simulink model "FrameStructTest"  (R2022b)
settings: Solver=VariableStepAuto  StartTime=0.0  StopTime=0.01  RelTol=1e-3
model workspace (MAT data in the model file):
  f_s : Simulink.Parameter (value not decoded)
symbols that are objects in the model workspace (value not decoded): f_s
libraries: simulink x24, hdlsllib x14, dspsigops x8, commdigbbndapm x3, dsphdlfiltering2 x2, commfilt2 x2, commdigbbndpm3 x2, commrandsrc3 x1
(part 2 of 2)

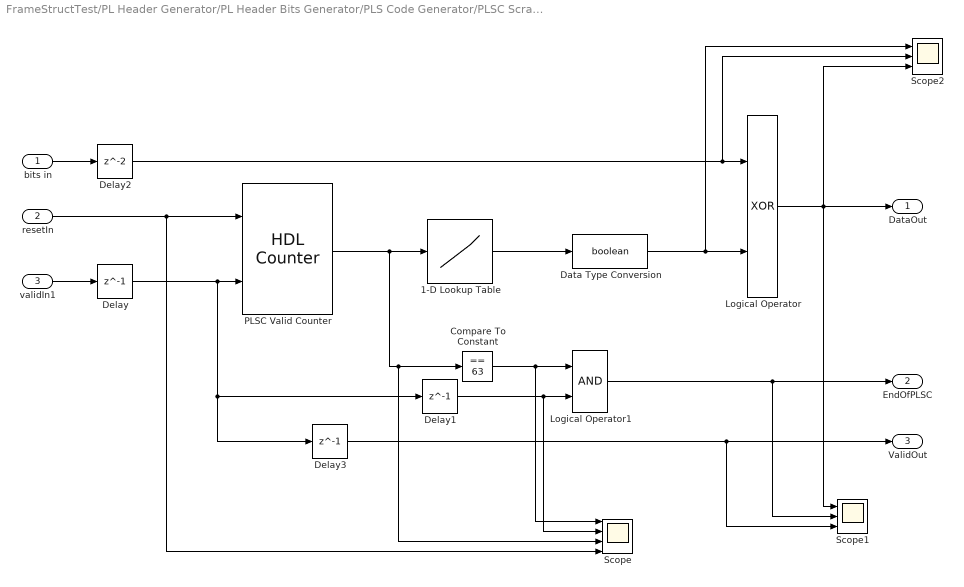
== system FrameStructTest/PL Header Generator/PL Header Bits Generator/PLS Code Generator/PLSC Scrambler ==
  bits in : Inport
  resetIn : Inport  Port=2
  validIn1 : Inport  Port=3
  1-D Lookup Table : Lookup_n-D  NumberOfTableDimensions=1  LookupTableObject=''  BreakpointsSpecification=Even spacing  BreakpointsForDimension1=[-5:5]  BreakpointsForDimension1FirstPoint=0  BreakpointsForDimension2FirstPoint=10  BreakpointsForDimension2Spacing=12  IndexSearchMethod=Evenly spaced points  Table=[1 0 1 1 1 1 0 0 0 0 0 1 0 0 0 1 1 0 0 0 0 0 0 0 1 0 1 0 0 1 0 1 0 1 0 1 0 0 0 1 0 1 1 1 0 1 1 1 0 1 0 1 1 1 0 0 1 0 0 1 1 1 0 1 1 0 0 0 0 1 0 1 1 0 0 0 1 1 1 1 1 1 0 1 1 0 1 0 1 1 0 0 1 1 0 1 1 0 1 1 1 0 0 0 0 1 1 1 0 0 0 1 1 0 1 0 1 0 0 1 1 1 1 1 0 0 0 1 0 0 0 0 1 1 0 0 1 0 1 0 0 0 0 0 0 1 1 1 1 0 1 1 1 1]  InterpMethod=Flat  DiagnosticForOutOfRangeInput=Error  InternalRulePriority=Speed  RndMeth=Simplest
  Compare To Constant : simulink/Logic and Bit Operations/Compare To Constant  relop===  const=63  OutDataTypeStr=boolean
  Data Type Conversion : DataTypeConversion  OutDataTypeStr=boolean  SaturateOnIntegerOverflow=off  RndMeth=Floor
  Delay : Delay  DelayLength=1
  Delay1 : Delay  DelayLength=1
  Delay2 : Delay
  Delay3 : Delay  DelayLength=1
  Logical Operator : Logic  Operator=XOR  AllPortsSameDT=off  OutDataTypeStr=boolean
  Logical Operator1 : Logic  AllPortsSameDT=off  OutDataTypeStr=boolean
  PLSC Valid Counter : hdlsllib/Sources/HDL Counter  CountType=Count limited  CountInit=0  CountStep=1  CountMax=154-1  CountFromType=Initial value  CountFrom=0  CountResetPort=on  CountLoadPort=off  CountEnbPort=on  CountDirPort=off  CountHitOutputPort=off  CountDataType=Unsigned  CountWordLen=8  CountFracLen=0  CountSampTime=1
  Scope : Scope  NumInputPorts=4
  Scope1 : Scope  NumInputPorts=3
  Scope2 : Scope  NumInputPorts=3
  DataOut : Outport
  EndOfPLSC : Outport  Port=2
  ValidOut : Outport  Port=3
  wires:
  PLSC Valid Counter/1 -> Scope/3, Compare To Constant/1, 1-D Lookup Table/1
  Data Type Conversion/1 -> Scope2/1, Logical Operator/2
  Logical Operator1/1 -> Scope1/2, EndOfPLSC/1
  Logical Operator/1 -> Scope2/3, Scope1/1, DataOut/1
  validIn1/1 -> Delay/1
  resetIn/1 -> Scope/4, PLSC Valid Counter/1
  Delay/1 -> Delay1/1, Delay3/1, PLSC Valid Counter/2
  Compare To Constant/1 -> Scope/1, Logical Operator1/1
  Delay1/1 -> Scope/2, Logical Operator1/2
  bits in/1 -> Delay2/1
  1-D Lookup Table/1 -> Data Type Conversion/1
  Delay2/1 -> Scope2/2, Logical Operator/1
  Delay3/1 -> Scope1/3, ValidOut/1

== system FrameStructTest/PL Header Generator/PL Header Bits Generator/PLS Code Generator/Serializer ==
  trigger : Inport
  coded bits : Inport  Port=2
  Compare To Constant : simulink/Logic and Bit Operations/Compare To Constant  relop===  const=1  OutDataTypeStr=boolean
  Compare To Constant1 : simulink/Logic and Bit Operations/Compare To Constant  relop=~=  const=1  OutDataTypeStr=boolean
  Constant : Constant  OutDataTypeStr=boolean  SampleTime=f_s/32*7
  Demux : Demux  Commented=on  Outputs=32
  HDL Counter : hdlsllib/Sources/HDL Counter  CountType=Count limited  CountInit=1  CountStep=1  CountMax=32  CountFromType=Initial value  CountFrom=1  CountResetPort=on  CountLoadPort=off  CountEnbPort=on  CountDirPort=off  CountHitOutputPort=off  CountDataType=Unsigned  CountWordLen=8  CountFracLen=0  CountSampTime=-1
  Logical Operator : Logic  AllPortsSameDT=off  OutDataTypeStr=boolean
  Logical Operator1 : Logic  AllPortsSameDT=off  OutDataTypeStr=boolean
  Logical Operator2 : Logic  Operator=OR  AllPortsSameDT=off  OutDataTypeStr=boolean
  Multiport Switch : MultiPortSwitch  Commented=on  Inputs=32  SaturateOnIntegerOverflow=off  InputSameDT=off
  NOT : Logic  Operator=NOT  IconShape=distinctive  AllPortsSameDT=off  OutDataTypeStr=boolean
  NOT1 : Logic  Operator=NOT  IconShape=distinctive  AllPortsSameDT=off  OutDataTypeStr=boolean
  Scope : Scope  NumInputPorts=4
  CodedBits1_7 : Outport
  startOut : Outport  Port=2
  validOut : Outport  Port=3
  wires:
  HDL Counter/1 -> Compare To Constant1/1, Scope/3, Compare To Constant/1
  Constant/1 -> HDL Counter/2
  trigger/1 -> NOT1/1
  NOT/1 -> Logical Operator1/1
  NOT1/1 -> Logical Operator/1
  Logical Operator1/1 -> Logical Operator2/1, Scope/1, startOut/1
  Compare To Constant/1 -> Logical Operator/2, Logical Operator1/2
  Logical Operator/1 -> NOT/1, HDL Counter/1
  Compare To Constant1/1 -> Logical Operator2/2
  Logical Operator2/1 -> Scope/2, validOut/1
  Demux/27 -> Multiport Switch/28
  Demux/29 -> Multiport Switch/30
  Demux/23 -> Multiport Switch/24
  Demux/24 -> Multiport Switch/25
  Demux/32 -> Multiport Switch/33
  Demux/30 -> Multiport Switch/31
  Demux/25 -> Multiport Switch/26
  Multiport Switch/1 -> ?
  Demux/15 -> Multiport Switch/16
  Demux/22 -> Multiport Switch/23
  Demux/18 -> Multiport Switch/19
  Demux/13 -> Multiport Switch/14
  Demux/26 -> Multiport Switch/27
  Demux/16 -> Multiport Switch/17
  ? -> Multiport Switch/1
  Demux/11 -> Multiport Switch/12
  Demux/21 -> Multiport Switch/22
  Demux/31 -> Multiport Switch/32
  Demux/12 -> Multiport Switch/13
  Demux/9 -> Multiport Switch/10
  Demux/14 -> Multiport Switch/15
  Demux/2 -> Multiport Switch/3
  Demux/5 -> Multiport Switch/6
  Demux/6 -> Multiport Switch/7
  Demux/8 -> Multiport Switch/9
  Demux/20 -> Multiport Switch/21
  Demux/1 -> Multiport Switch/2
  Demux/19 -> Multiport Switch/20
  Demux/10 -> Multiport Switch/11
  Demux/3 -> Multiport Switch/4
  Demux/28 -> Multiport Switch/29
  Demux/17 -> Multiport Switch/18
  Demux/7 -> Multiport Switch/8
  Demux/4 -> Multiport Switch/5
  coded bits/1 -> Scope/4, CodedBits1_7/1

== system FrameStructTest/PL Header Generator/PL Header Bits Generator/SOF Generator/SOF Length Counter ==
  Trigger : Inport
  Constant : Constant  SampleTime=-1
  Data Type Conversion : DataTypeConversion  OutDataTypeStr=boolean  SaturateOnIntegerOverflow=off  RndMeth=Floor
  HDL Counter1 : hdlsllib/Sources/HDL Counter  CountType=Count limited  CountInit=0  CountStep=1  CountMax=25  CountFromType=Initial value  CountFrom=0  CountResetPort=on  CountLoadPort=off  CountEnbPort=on  CountDirPort=off  CountHitOutputPort=on  CountDataType=Unsigned  CountWordLen=8  CountFracLen=0  CountSampTime=1
  IsNonZero : simulink/Logic and Bit Operations/Compare To Zero  relop=~=  OutDataTypeStr=boolean
      settings: LibrarySourceBlock=|
      | simulink/Quick Insert/Logic and Bit
      | Operations/IsNonZero
  IsZero : simulink/Logic and Bit Operations/Compare To Zero  relop===  OutDataTypeStr=boolean
      settings: LibrarySourceBlock=|
      | simulink/Quick Insert/Logic and Bit
      | Operations/IsZero
  Logical Operator : Logic  AllPortsSameDT=off  OutDataTypeStr=boolean
  Logical Operator1 : Logic  AllPortsSameDT=off  OutDataTypeStr=boolean
  Logical Operator2 : Logic  Operator=OR  AllPortsSameDT=off  OutDataTypeStr=boolean
  NOT : Logic  Operator=NOT  IconShape=distinctive  AllPortsSameDT=off  OutDataTypeStr=boolean
  NOT1 : Logic  Operator=NOT  IconShape=distinctive  AllPortsSameDT=off  OutDataTypeStr=boolean
  Scope : Scope  Commented=on  NumInputPorts=3
  LUT address : Outport
  validOut : Outport  Port=2
  StartOfOSOF : Outport  Port=3
  wires:
  IsZero/1 -> Logical Operator1/2, Logical Operator/1
  Trigger/1 -> NOT/1
  Data Type Conversion/1 -> HDL Counter1/2
  Constant/1 -> Data Type Conversion/1
  NOT/1 -> Logical Operator/2
  Logical Operator/1 -> NOT1/1, HDL Counter1/1
  IsNonZero/1 -> Logical Operator2/2
  NOT1/1 -> Logical Operator1/1
  Logical Operator1/1 -> Scope/3, Logical Operator2/1, StartOfOSOF/1
  HDL Counter1/1 -> Scope/1, LUT address/1, IsNonZero/1, IsZero/1
  Logical Operator2/1 -> Scope/2, validOut/1

== system FrameStructTest/PL Header Generator/PL Header Bits Generator/PLS Code Generator/Biorthogonal code/Modulo-2 ==
  In1 : Inport
  Data Type Conversion : DataTypeConversion  OutDataTypeStr=boolean  SaturateOnIntegerOverflow=off  RndMeth=Floor
  Extract Bits : simulink/Logic and Bit Operations/Extract Bits  bitsToExtract=Range of bits  numBits=7  bitIdxRange=0  outScalingMode=Treat bit field as an integer
  coded bits : Outport
  wires:
  In1/1 -> Extract Bits/1
  Extract Bits/1 -> Data Type Conversion/1
  Data Type Conversion/1 -> coded bits/1
